simulink model "A2c"  (R2024a)
settings: Solver=ode113  StartTime=0.0  StopTime=100  RelTol=1e-3
settings Model: Creator=Flipper  LastModifiedBy=Flipper

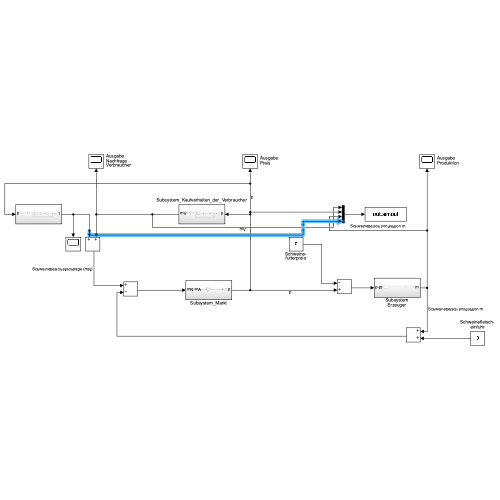
[thumbnail: Simulink's stored preview of the top-level diagram]
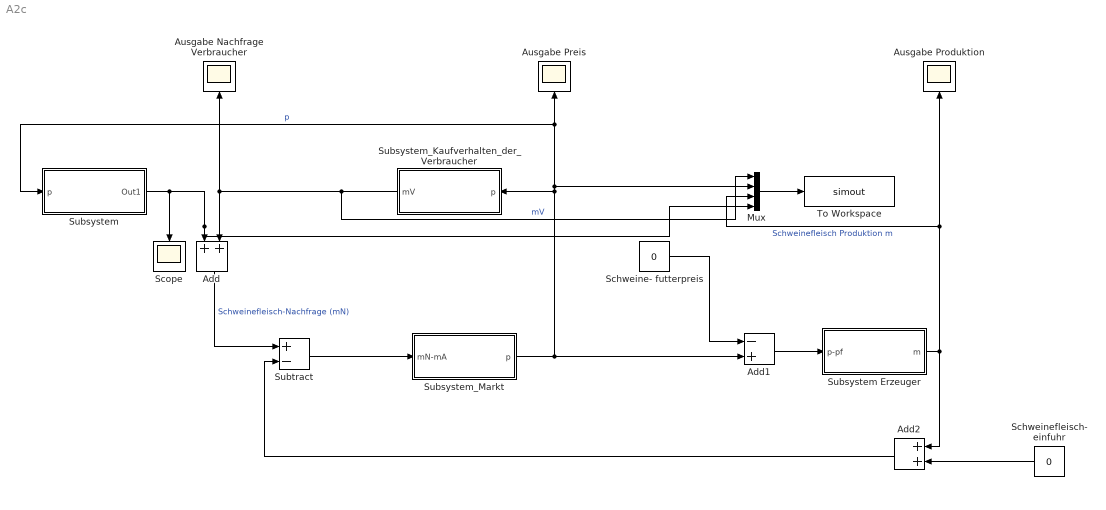
== system A2c ==
  Add : Sum
  Add1 : Sum  Inputs=-+
  Add2 : Sum
  Ausgabe Nachfrage Verbraucher : Scope
  Ausgabe Preis : Scope
  Ausgabe Produktion : Scope
  Mux : Mux
  Schweine- futterpreis : Constant  Value=0
  Schweinefleisch- einfuhr : Constant  Value=0
  Scope : Scope
  Subsystem : Subsystem
  Subsystem Erzeuger : Subsystem
  Subsystem_Kaufverhalten_der_Verbraucher : Subsystem
  Subsystem_Markt : Subsystem
  Subtract : Sum  Inputs=+-
  To Workspace : ToWorkspace  VariableName=simout  SaveFormat=Timeseries  SampleTime=-1
  wires:
  Add1/1 -> Subsystem Erzeuger/1(p-pf)
  Subtract/1 -> Subsystem_Markt/1(mN-mA)
  Schweinefleisch- einfuhr/1 -> Add2/2
  Schweine- futterpreis/1 -> Add1/1
  Add2/1 -> Subtract/2
  Subsystem_Kaufverhalten_der_Verbraucher/1(mV) -> Mux/1, Ausgabe Nachfrage Verbraucher/1, Add/2  "mV"
  Subsystem Erzeuger/1(m) -> Ausgabe Produktion/1, Mux/3, Add2/1  "Schweinefleisch Produktion m"
  Add/1 -> Subtract/1  "Schweinefleisch-Nachfrage (mN)"
  Subsystem_Markt/1(p) -> Subsystem/1(p), Ausgabe Preis/1, Mux/2, Subsystem_Kaufverhalten_der_Verbraucher/1(p), Add1/2  "p"
  Mux/1 -> To Workspace/1
  Subsystem/1(Out1) -> Scope/1, Mux/4, Add/1

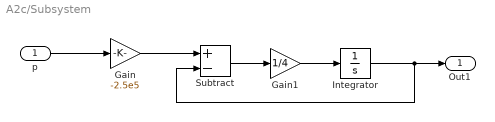
== system A2c/Subsystem ==
  p : Inport
  Gain : Gain  Gain=-2.5e5
  Gain1 : Gain  Gain=1/4
  Integrator : Integrator
  Subtract : Sum  Inputs=+-
  Out1 : Outport
  wires:
  Gain/1 -> Subtract/1
  Subtract/1 -> Gain1/1
  Gain1/1 -> Integrator/1
  Integrator/1 -> Subtract/2, Out1/1
  p/1 -> Gain/1

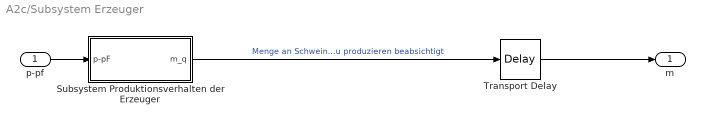
== system A2c/Subsystem Erzeuger ==
  p-pf : Inport
  Subsystem Produktionsverhalten der Erzeuger : Subsystem
  Transport Delay : TransportDelay  DelayTime=10
  m : Outport
  wires:
  p-pf/1 -> Subsystem Produktionsverhalten der Erzeuger/1(p-pF)
  Subsystem Produktionsverhalten der Erzeuger/1(m_q) -> Transport Delay/1  "Menge an Schweinefleisch, die der Erzeuger zu produzieren beabsichtigt"
  Transport Delay/1 -> m/1

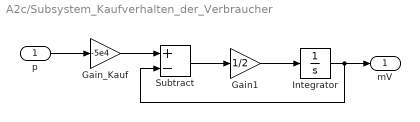
== system A2c/Subsystem_Kaufverhalten_der_Verbraucher ==
  p : Inport
  Gain1 : Gain  Gain=1/2
  Gain_Kauf : Gain  Gain=-5e4
  Integrator : Integrator  InitialCondition=-5e4
  Subtract : Sum  Inputs=+-
  mV : Outport
  wires:
  p/1 -> Gain_Kauf/1
  Gain_Kauf/1 -> Subtract/1
  Subtract/1 -> Gain1/1
  Gain1/1 -> Integrator/1
  Integrator/1 -> Subtract/2, mV/1

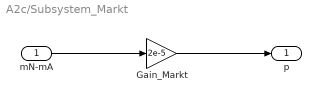
== system A2c/Subsystem_Markt ==
  mN-mA : Inport
  Gain_Markt : Gain  Gain=2e-5
  p : Outport
  wires:
  mN-mA/1 -> Gain_Markt/1
  Gain_Markt/1 -> p/1

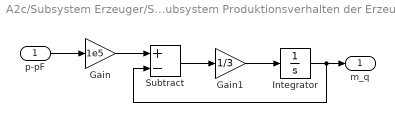
== system A2c/Subsystem Erzeuger/Subsystem Produktionsverhalten der Erzeuger ==
  p-pF : Inport
  Gain : Gain  Gain=1e5
  Gain1 : Gain  Gain=1/3
  Integrator : Integrator
  Subtract : Sum  Inputs=+-
  m_q : Outport
  wires:
  p-pF/1 -> Gain/1
  Gain/1 -> Subtract/1
  Subtract/1 -> Gain1/1
  Integrator/1 -> Subtract/2, m_q/1
  Gain1/1 -> Integrator/1
